simulink model "Hydrogen_platform"  (R2024b)
settings: Solver=VariableStepAuto  StartTime=0.0  StopTime=10.0  FixedStep=0.001  RelTol=1e-3
(part 2 of 2)

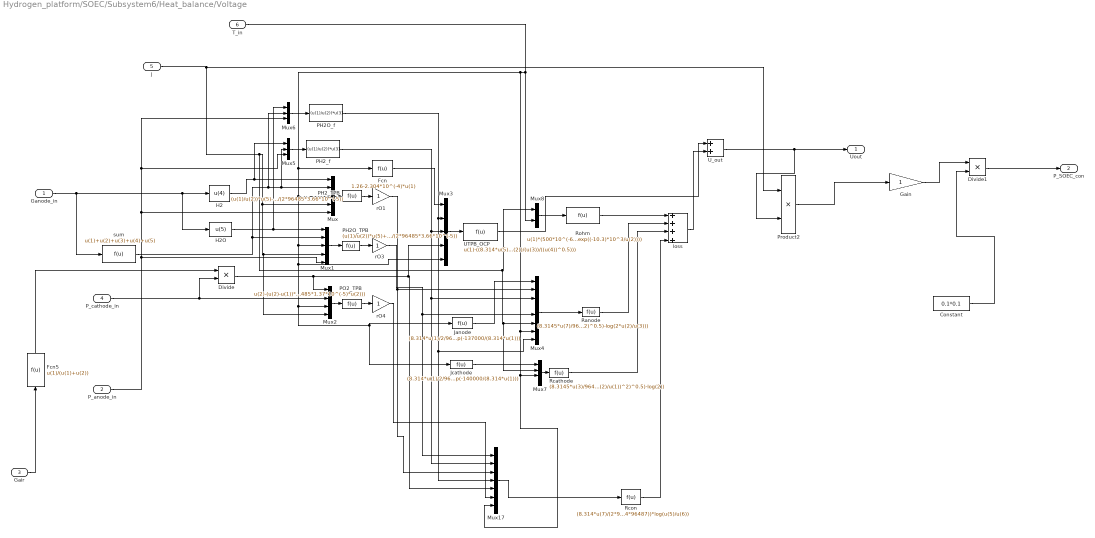
== system Hydrogen_platform/SOEC/Subsystem6/Heat_balance/Voltage ==
  Ganode_in : Inport
  P_anode_in : Inport  Port=2
  Gair : Inport  Port=3
  P_cathode_in : Inport  Port=4
  j : Inport  Port=5
  T_in : Inport  Port=6
  Constant : Constant  Value=0.1*0.1
  Divide : Product  Inputs=**
  Divide1 : Product  Inputs=**
  Fcn : Fcn  Expr=1.26-2.304*10^(-4)*u(1)
  Fcn5 : Fcn  Expr=u(1)/(u(1)+u(2))
  Gain : Gain
  H2 : Fcn  Expr=u(4)
  H2O : Fcn  Expr=u(5)
  Janode : Fcn  Expr=(8.314*u(1)/2/96485)*2.35*10^11*exp(-137000/(8.314*u(1)))
  Jcathode : Fcn  Expr=(8.314*u(1)/2/96485)*6.54*10^11*exp(-140000/(8.314*u(1)))
  Mux : Mux  Inputs=5
  Mux1 : Mux  Inputs=5
  Mux17 : Mux  Inputs=7
  Mux2 : Mux
  Mux3 : Mux  Inputs=5
  Mux4 : Mux  Inputs=8
  Mux5 : Mux  Inputs=3
  Mux6 : Mux  Inputs=3
  Mux7 : Mux
  Mux8 : Mux  Inputs=2
  PH2O_TPB : Fcn  Expr=(u(1)/u(2))*u(5)+8.314*u(3)*500*10^(-6)*u(4)/(2*96485*3.66*10^(-5))
  PH2O_f : Fcn  Expr=(u(1)/u(2))*u(3)
  PH2_TPB : Fcn  Expr=(u(1)/u(2))*u(5)-8.314*u(3)*500*10^(-6)*u(4)/(2*96485*3.66*10^(-5))
  PH2_f : Fcn  Expr=(u(1)/u(2))*u(3)
  PO2_TPB : Fcn  Expr=u(2)-(u(2)-u(1))*exp(8.314*u(3)*50*10^(-6)*u(4)/(4*96485*1.37*10^(-5)*u(2)))
  Product2 : Product
  Ranode : Fcn  Expr=(8.3145*u(7)/96485)*(log(u(6)/u(1)+(4*(u(2)/u(3))*(u(5)/u(8))+(u(6)/u(1))^2)^0.5)-log(2*u(2)/u(3)))
  Rcathode : Fcn  Expr=(8.3145*u(3)/96485)*(log(u(2)/u(1)+(4+(u(2)/u(1))^2)^0.5)-log(2))
  Rcon : Fcn  Expr=(8.314*u(7)/(2*96487))*log((u(1)*u(2))/(u(3)*u(4)))+(8.314*u(7)/(4*96487))*log(u(5)/u(6))
  Rohm : Fcn  Expr=u(1)*(500*10^(-6)/(8*10^4)+50*10^(-6)/(8.4*10^3)+20*10^(-6)/(33.4*10^3*exp((-10.3)*10^3/u(2))))
  UTPB_OCP : Fcn  Expr=u(1)-((8.314*u(5)/2/96485)*log((u(2))/(u(3))/((u(4))^0.5)))
  U_out : Sum
  loss : Sum  Inputs=++++
  rO1 : Gain
  rO3 : Gain
  rO4 : Gain
  sum : Fcn  Expr=u(1)+u(2)+u(3)+u(4)+u(5)
  Uout : Outport  VectorParamsAs1DForOutWhenUnconnected=off
  P_SOEC_con : Outport  Port=2  VectorParamsAs1DForOutWhenUnconnected=off
  wires:
  Ganode_in/1 -> H2O/1, H2/1, sum/1
  H2/1 -> Mux5/1, Mux/1
  sum/1 -> Mux1/2, Mux6/2, Mux5/2, Mux/2
  Mux/1 -> PH2_TPB/1
  j/1 -> Mux7/2, Mux4/6, Mux8/1, Mux2/4, Mux1/4, Mux/4, Product2/1
  Mux1/1 -> PH2O_TPB/1
  H2O/1 -> Mux6/1, Mux1/1
  Mux2/1 -> PO2_TPB/1
  Fcn/1 -> Mux3/1
  PH2O_TPB/1 -> rO3/1
  PH2_TPB/1 -> rO1/1
  PO2_TPB/1 -> rO4/1
  Mux3/1 -> UTPB_OCP/1
  Mux5/1 -> PH2_f/1
  Mux6/1 -> PH2O_f/1
  Mux8/1 -> Rohm/1
  Rohm/1 -> loss/1
  UTPB_OCP/1 -> U_out/1
  U_out/1 -> Product2/2, Uout/1
  Product2/1 -> Gain/1
  Gair/1 -> Fcn5/1
  P_cathode_in/1 -> Divide/2, Mux2/2
  P_anode_in/1 -> Mux1/5, Mux/5, Mux5/3, Mux6/3
  Rcon/1 -> loss/4
  Fcn5/1 -> Divide/1
  Janode/1 -> Mux4/1
  Ranode/1 -> loss/2
  Mux7/1 -> Rcathode/1
  Jcathode/1 -> Mux7/1
  Rcathode/1 -> loss/3
  rO3/1 -> Mux17/1, Mux4/5
  PH2_f/1 -> Mux3/3, Mux17/2, Mux4/3
  Divide/1 -> Mux17/5, Mux3/4, Mux2/1
  rO1/1 -> Mux17/3, Mux4/2
  PH2O_f/1 -> Mux3/2, Mux17/4, Mux4/8
  rO4/1 -> Mux17/6
  Divide1/1 -> P_SOEC_con/1
  Mux4/1 -> Ranode/1
  Mux17/1 -> Rcon/1
  Gain/1 -> Divide1/1
  Constant/1 -> Divide1/2
  T_in/1 -> Mux8/2, Fcn/1, Mux/3, Mux1/3, Mux3/5, Jcathode/1, Janode/1, Mux2/3, Mux4/7, Mux7/3, Mux17/7
  loss/1 -> U_out/2

== system Hydrogen_platform/SOEC/Subsystem6/Heat_balance/Heat/Cp3 ==
  T_cool_out : Inport
  O2 : Inport  Port=2
  h2 : Inport  Port=3
  Add : Sum  Inputs=++-
  Enthalpy of formation of Oxygen : Fcn  Expr=3.46428571428576e-06*u(1)^2+0.0279630952380952*u(1)-8.69654761904760
  Enthalpy of formation of hydrogen : Fcn  Expr=7.20238095238088e-07*u(1)^2+0.0285172619047619*u(1)-8.56458333333334
  Enthalpy of formation of steam : Fcn  Expr=5.41666666666615e-06*u(1)^2+0.0302750000000008*u(1)-251.511666666667
  Gain1 : Gain  Gain=1000
  Product1 : Product
  Product4 : Product
  Product5 : Product
  Reaction Thermal : Outport  VectorParamsAs1DForOutWhenUnconnected=off
  wires:
  T_cool_out/1 -> Enthalpy of formation of hydrogen/1, Enthalpy of formation of steam/1, Enthalpy of formation of Oxygen/1
  Enthalpy of formation of hydrogen/1 -> Product4/1
  Enthalpy of formation of Oxygen/1 -> Product5/1
  O2/1 -> Product5/2
  Add/1 -> Gain1/1
  Product4/1 -> Add/1
  Product5/1 -> Add/2
  Enthalpy of formation of steam/1 -> Product1/1
  h2/1 -> Product4/2, Product1/2
  Product1/1 -> Add/3
  Gain1/1 -> Reaction Thermal/1

== system Hydrogen_platform/SOEC/Subsystem6/Heat_balance/Heat/Fuel_in ==
  T_cool_out : Inport
  CH4 : Inport  Port=2
  CO : Inport  Port=3
  CO2 : Inport  Port=4
  H2 : Inport  Port=5
  H2O : Inport  Port=6
  Add : Sum  Inputs=+++++
  Product{,1..3,6} (5 alike) : Product
  cpCH4_T : Fcn  Expr=(14.1555+0.0755466*u(1)-0.0000180032*u(1)^2)*u(1)
  cpCO2_T : Fcn  Expr=(26.0167+0.0435259*u(1)-0.0000148422*u(1)^2)*u(1)
  cpCO_T : Fcn  Expr=(26.8742+0.0069710*u(1)-0.0000008206*u(1)^2)*u(1)
  cpH20_T : Fcn  Expr=(30.3794+0.0096212*u(1)-0.0000011848*u(1)^2)*u(1)
  cpH2_T : Fcn  Expr=(29.08-0.00084*u(1)+0.000002*u(1)^2)*u(1)
  energy_cool_out : Outport  VectorParamsAs1DForOutWhenUnconnected=off
  wires:
  T_cool_out/1 -> cpH20_T/1, cpCO2_T/1, cpCO_T/1, cpH2_T/1, cpCH4_T/1
  cpCH4_T/1 -> Product/1
  CH4/1 -> Product/2
  cpH2_T/1 -> Product1/1
  H2/1 -> Product1/2
  cpCO_T/1 -> Product2/1
  CO/1 -> Product2/2
  cpCO2_T/1 -> Product3/1
  CO2/1 -> Product3/2
  cpH20_T/1 -> Product6/1
  H2O/1 -> Product6/2
  Product/1 -> Add/1
  Product1/1 -> Add/2
  Product2/1 -> Add/3
  Product3/1 -> Add/4
  Add/1 -> energy_cool_out/1
  Product6/1 -> Add/5

== system Hydrogen_platform/SOEC/Subsystem6/Heat_balance/Heat/air_in ==
  T_cool_out : Inport
  O2 : Inport  Port=2
  N2 : Inport  Port=3
  Add : Sum
  Product4 : Product
  Product5 : Product
  cpN2_T : Fcn  Expr=(27.32+(6.226*10^(-3))*u(1)-(9.502*10^(-7))*u(1)^2)*u(1)
  cpO2_T : Fcn  Expr=(25.8911+0.01299*u(1)-0.0000038644*u(1)^2)*u(1)
  energy_cool_out : Outport  VectorParamsAs1DForOutWhenUnconnected=off
  wires:
  T_cool_out/1 -> cpO2_T/1, cpN2_T/1
  cpN2_T/1 -> Product4/1
  N2/1 -> Product4/2
  cpO2_T/1 -> Product5/1
  O2/1 -> Product5/2
  Add/1 -> energy_cool_out/1
  Product4/1 -> Add/1
  Product5/1 -> Add/2

== system Hydrogen_platform/SOEC/Subsystem6/Heat_balance/Heat/air_out ==
  T_cool_out : Inport
  O2 : Inport  Port=2
  N2 : Inport  Port=3
  Add : Sum
  Product4 : Product
  Product5 : Product
  cpN2_T : Fcn  Expr=(27.32+(6.226*10^(-3))*u(1)-(9.502*10^(-7))*u(1)^2)*u(1)
  cpO2_T : Fcn  Expr=(25.8911+0.01299*u(1)-0.0000038644*u(1)^2)*u(1)
  energy_cool_out : Outport  VectorParamsAs1DForOutWhenUnconnected=off
  wires:
  T_cool_out/1 -> cpO2_T/1, cpN2_T/1
  cpN2_T/1 -> Product4/1
  N2/1 -> Product4/2
  cpO2_T/1 -> Product5/1
  O2/1 -> Product5/2
  Add/1 -> energy_cool_out/1
  Product4/1 -> Add/1
  Product5/1 -> Add/2

== system Hydrogen_platform/SOEC/Subsystem6/Heat_balance/Heat/fuel_out ==
  T_cool_out : Inport
  CH4 : Inport  Port=2
  CO : Inport  Port=3
  CO2 : Inport  Port=4
  H2 : Inport  Port=5
  H2O : Inport  Port=6
  Add : Sum  Inputs=+++++
  Product{,1..3,6} (5 alike) : Product
  cpCH4_T : Fcn  Expr=(14.1555+0.0755466*u(1)-0.0000180032*u(1)^2)*u(1)
  cpCO2_T : Fcn  Expr=(26.0167+0.0435259*u(1)-0.0000148422*u(1)^2)*u(1)
  cpCO_T : Fcn  Expr=(26.8742+0.0069710*u(1)-0.0000008206*u(1)^2)*u(1)
  cpH20_T : Fcn  Expr=(30.3794+0.0096212*u(1)-0.0000011848*u(1)^2)*u(1)
  cpH2_T : Fcn  Expr=(29.08-0.00084*u(1)+0.000002*u(1)^2)*u(1)
  energy_cool_out : Outport  VectorParamsAs1DForOutWhenUnconnected=off
  wires:
  T_cool_out/1 -> cpH20_T/1, cpCO2_T/1, cpCO_T/1, cpH2_T/1, cpCH4_T/1
  cpCH4_T/1 -> Product/1
  CH4/1 -> Product/2
  cpH2_T/1 -> Product1/1
  H2/1 -> Product1/2
  cpCO_T/1 -> Product2/1
  CO/1 -> Product2/2
  cpCO2_T/1 -> Product3/1
  CO2/1 -> Product3/2
  cpH20_T/1 -> Product6/1
  H2O/1 -> Product6/2
  Product/1 -> Add/1
  Product1/1 -> Add/2
  Product2/1 -> Add/3
  Product3/1 -> Add/4
  Add/1 -> energy_cool_out/1
  Product6/1 -> Add/5
